simulink model "quad_system_1"  (R2023a)
settings: Solver=VariableStepAuto  StartTime=0.0  StopTime=30  RelTol=1e-7
InitFcn:
  | % Init parameters
  | ax = 0; ay = 0; az = 0;
  | a_theta = 0; a_phi = 0; a_psi = 0;
  | m = 1;
  | J_phi = 1;
  | J_psi = 1;
  | C = 1;
  | L = 1;
  | J_theta = 1;
  | g = 9.81;
  | alpha = 0.9;
  | K = alpha*g;
  | 
  | %Controller for Z/phi
  | k_11 = 100;
  | k_21 = 100;
  | k_12 = 1;
  | k_22 = 1;
  | 
  | %Controller for X/Y
  | k31=100;
  | k41=100;
  | k51=100;
  | k61=10;
  | 
  | k32=100;
  | k42=100;
  | k52=100;
  | k62=10;
  | % k31=1000;
  | % k41=100;
  | % k51=100;
  | % k61=1;
  | %
  | % k32=1000;
  | % k42=100;
  | % k52=100;
  | % k62=1;
  | 
  | J = [0 -1; 1 0];
settings Model: Creator=Dell  LastModifiedBy=Dell
settings DebuggingCC: UnconnectedInputMsg=warning  UnconnectedOutputMsg=warning  UnconnectedLineMsg=warning
settings ModelReferenceCC: EnableRefExpFcnMdlSchedulingChecks=on
settings RTWCC: DLArmComputeVersion=19.05

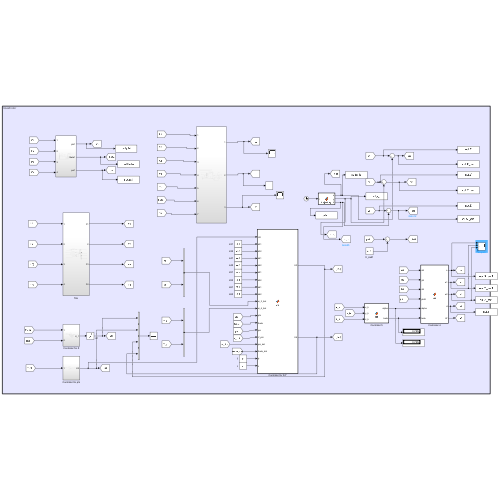
[thumbnail: Simulink's stored preview of the top-level diagram]
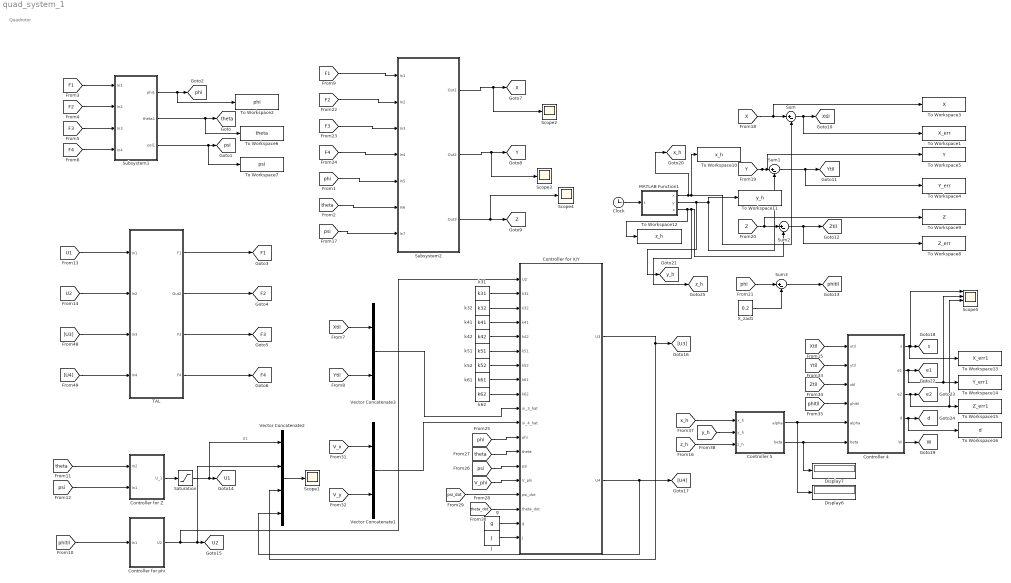
== system quad_system_1 ==
  note: Quadrotor
  Clock : Clock
  Controller 4 : MATLAB Function  TreatAsAtomicUnit=on
  Controller 5 : MATLAB Function  TreatAsAtomicUnit=on
  Controller for X/Y : MATLAB Function  TreatAsAtomicUnit=on
  Controller for Z : Subsystem
  Controller for phi : Subsystem
  Display6 : Display
  Display7 : Display
  J : Constant  Value=J
  MATLAB Function1 : MATLAB Function  TreatAsAtomicUnit=on
  Saturation : Saturate  UpperLimit=K  LowerLimit=-K
  Scope{1..4} (4 alike) : Scope
  Scope5 : Scope  NumInputPorts=4
  Subsystem1 : Subsystem
  Subsystem2 : Subsystem
  Sum{,1..3} (4 alike) : Sum  Inputs=|+-
  TAL : Subsystem
  To Workspace1 : ToWorkspace  VariableName=X_err  SaveFormat=Timeseries  SampleTime=-1
  To Workspace10 : ToWorkspace  VariableName=x_h  SaveFormat=Timeseries  SampleTime=-1
  To Workspace11 : ToWorkspace  VariableName=y_h  SaveFormat=Timeseries  SampleTime=-1
  To Workspace12 : ToWorkspace  VariableName=z_h  SaveFormat=Timeseries  SampleTime=-1
  To Workspace13 : ToWorkspace  VariableName=X_err1  SaveFormat=Timeseries  SampleTime=-1
  To Workspace14 : ToWorkspace  VariableName=Y_err1  SaveFormat=Timeseries  SampleTime=-1
  To Workspace15 : ToWorkspace  VariableName=Z_err1  SaveFormat=Timeseries  SampleTime=-1
  To Workspace16 : ToWorkspace  VariableName=d  SaveFormat=Timeseries  SampleTime=-1
  To Workspace2 : ToWorkspace  VariableName=phi  SaveFormat=Timeseries  SampleTime=-1
  To Workspace3 : ToWorkspace  VariableName=X  SaveFormat=Timeseries  SampleTime=-1
  To Workspace4 : ToWorkspace  VariableName=Y_err  SaveFormat=Timeseries  SampleTime=-1
  To Workspace5 : ToWorkspace  VariableName=Y  SaveFormat=Timeseries  SampleTime=-1
  To Workspace6 : ToWorkspace  VariableName=theta  SaveFormat=Timeseries  SampleTime=-1
  To Workspace7 : ToWorkspace  VariableName=psi  SaveFormat=Timeseries  SampleTime=-1
  To Workspace8 : ToWorkspace  VariableName=Z_err  SaveFormat=Timeseries  SampleTime=-1
  To Workspace9 : ToWorkspace  VariableName=Z  SaveFormat=Timeseries  SampleTime=-1
  Vector Concatenate1 : Concatenate
  Vector Concatenate2 : Concatenate  NumInputs=4
  Vector Concatenate3 : Concatenate
  X_zad1 : Constant  Value=0.2
  g : Constant  Value=g
  k31 : Constant  Value=k31
  k32 : Constant  Value=k32
  k41 : Constant  Value=k41
  k42 : Constant  Value=k42
  k51 : Constant  Value=k51
  k52 : Constant  Value=k52
  k61 : Constant  Value=k61
  k62 : Constant  Value=k62
  tag scope: F1=global, F2=global, F3=global, F4=global, U1=global, U2=global, W=global, X=global, Xtil=global, Y=global, Ytil=global, Z=global, Ztil=global, d=global, e1=global, e2=global, phi=global, phitil=global, psi=global, s=global, theta=global, x_h=global, y_h=global, z_h=global
  wires:
  Subsystem1/1(phi1) -> To Workspace2/1, [phi]
  [phi] -> Subsystem2/5(In5)
  [theta] -> Subsystem2/6(In6)
  [psi] -> Subsystem2/7(In7)
  Subsystem2/2(Out2) -> Scope3/1, [Y]
  Subsystem2/3(Out3) -> Scope4/1, [Z]
  TAL/1(F1) -> [F1]
  TAL/2(Out2) -> [F2]
  TAL/3(F3) -> [F3]
  TAL/4(F4) -> [F4]
  [Z] -> To Workspace9/1, Sum2/1
  [Y] -> To Workspace5/1, Sum1/1
  X_zad1/1 -> Sum3/2
  [phi] -> Sum3/1
  Sum/1 -> To Workspace1/1, [Xtil]
  Sum1/1 -> To Workspace4/1, [Ytil]
  Sum3/1 -> [phitil]
  Sum2/1 -> To Workspace8/1, [Ztil]
  [phitil] -> Controller for phi/1(In1)
  Controller for phi/1(U2) -> Controller for X/Y/1(U2), Vector Concatenate2/2, [U2]
  Controller for Z/1(U_1) -> Saturation/1
  Saturation/1 -> Vector Concatenate2/1, [U1]  "U1"
  [F1] -> Subsystem1/1(In1)
  [F2] -> Subsystem1/2(In2)
  [F3] -> Subsystem1/3(In3)
  [F4] -> Subsystem1/4(In4)
  [F1] -> Subsystem2/1(In1)
  [F2] -> Subsystem2/2(In2)
  [F3] -> Subsystem2/3(In3)
  [F4] -> Subsystem2/4(In4)
  Controller for X/Y/1(U3) -> Vector Concatenate2/3, [U3]
  Controller for X/Y/2(U4) -> Vector Concatenate2/4, [U4]
  [Xtil] -> Vector Concatenate3/1
  [Ytil] -> Vector Concatenate3/2
  [phi] -> Controller for X/Y/12(phi)
  [theta] -> Controller for X/Y/13(theta)
  [psi] -> Controller for X/Y/14(psi)
  [V_phi] -> Controller for X/Y/15(V_phi)
  [psi_dot] -> Controller for X/Y/16(psi_dot)
  [theta_dot] -> Controller for X/Y/17(theta_dot)
  k31/1 -> Controller for X/Y/2(k31)
  k32/1 -> Controller for X/Y/3(k32)
  k41/1 -> Controller for X/Y/4(k41)
  k42/1 -> Controller for X/Y/5(k42)
  g/1 -> Controller for X/Y/18(g)
  J/1 -> Controller for X/Y/19(J)
  Vector Concatenate3/1 -> Controller for X/Y/10(xi_3_hat)
  Vector Concatenate1/1 -> Controller for X/Y/11(xi_4_hat)
  [V_x] -> Vector Concatenate1/1
  [V_y] -> Vector Concatenate1/2
  [U3] -> TAL/3(In3)
  [U4] -> TAL/4(In4)
  [U1] -> TAL/1(In1)
  [U2] -> TAL/2(In2)
  Subsystem2/1(Out1) -> Scope2/1, [X]
  [theta] -> Controller for Z/1(In2)
  [psi] -> Controller for Z/2(In1)
  Vector Concatenate2/1 -> Scope1/1
  [X] -> To Workspace3/1, Sum/1
  k51/1 -> Controller for X/Y/6(k51)
  k52/1 -> Controller for X/Y/7(k52)
  k61/1 -> Controller for X/Y/8(k61)
  k62/1 -> Controller for X/Y/9(k62)
  Subsystem1/2(theta1) -> To Workspace6/1, [theta]
  Subsystem1/3(psi1) -> To Workspace7/1, [psi]
  Clock/1 -> MATLAB Function1/1(t)
  MATLAB Function1/1(x) -> [x_h], To Workspace10/1, Sum/2
  MATLAB Function1/2(y) -> [y_h], Sum1/2, To Workspace11/1
  MATLAB Function1/3(z) -> To Workspace12/1, [z_h], Sum2/2
  Controller 4/3(e2) -> Scope5/3, To Workspace15/1, [e2]
  [Ytil] -> Controller 4/2(ytil)
  [Xtil] -> Controller 4/1(xtil)
  [x_h] -> Controller 5/1(x_h)
  Controller 4/4(d) -> To Workspace16/1, [d]
  [Ztil] -> Controller 4/3(ztil)
  [z_h] -> Controller 5/3(z_h)
  Controller 4/2(e1) -> Scope5/2, To Workspace14/1, [e1]
  [phitil] -> Controller 4/4(phitil)
  [y_h] -> Controller 5/2(y_h)
  Controller 4/5(W) -> [W]
  Controller 5/2(beta) -> Controller 4/6(beta), Display7/1
  Controller 5/1(alpha) -> Display6/1, Controller 4/5(alpha)
  Controller 4/1(s) -> Scope5/1, [s], To Workspace13/1

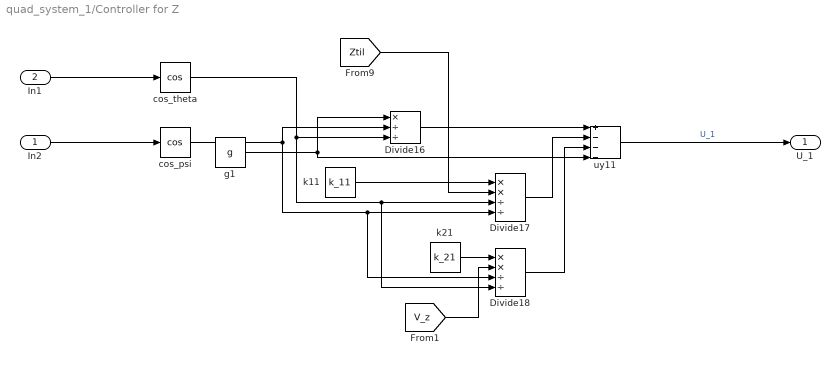
== system quad_system_1/Controller for Z ==
  In2 : Inport
  In1 : Inport  Port=2
  Divide16 : Product  Inputs=*//
  Divide17 : Product  Inputs=**//
  Divide18 : Product  Inputs=**//
  cos_psi : Trigonometry  Operator=cos
  cos_theta : Trigonometry  Operator=cos
  g1 : Constant  Value=g
  k11 : Constant  Value=k_11
  k21 : Constant  Value=k_21
  uy11 : Sum  Inputs=+---
  U_1 : Outport
  wires:
  k11/1 -> Divide17/1
  g1/1 -> uy11/4, Divide16/1
  Divide16/1 -> uy11/1
  k21/1 -> Divide18/1
  Divide18/1 -> uy11/3
  Divide17/1 -> uy11/2
  cos_theta/1 -> Divide16/3, Divide18/4, Divide17/3
  [Ztil] -> Divide17/2
  cos_psi/1 -> Divide16/2, Divide18/3, Divide17/4
  uy11/1 -> U_1/1  "U_1"
  In1/1 -> cos_theta/1
  In2/1 -> cos_psi/1
  [V_z] -> Divide18/2

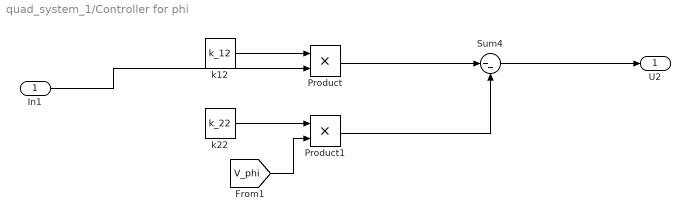
== system quad_system_1/Controller for phi ==
  In1 : Inport
  Product : Product
  Product1 : Product
  Sum4 : Sum  Inputs=|--
  k12 : Constant  Value=k_12
  k22 : Constant  Value=k_22
  U2 : Outport
  wires:
  In1/1 -> Product/2
  Sum4/1 -> U2/1
  k22/1 -> Product1/1
  k12/1 -> Product/1
  Product/1 -> Sum4/1
  Product1/1 -> Sum4/2
  [V_phi] -> Product1/2

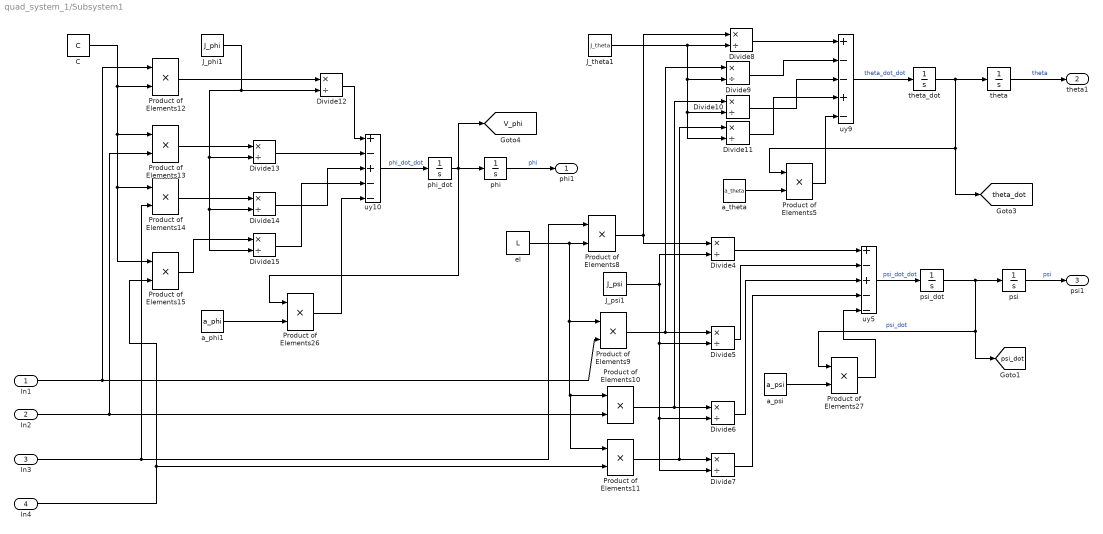
== system quad_system_1/Subsystem1 ==
  In1 : Inport
  In2 : Inport  Port=2
  In3 : Inport  Port=3
  In4 : Inport  Port=4
  C : Constant  Value=C
  Divide{4..15} (12 alike) : Product  Inputs=*/
  J_phi1 : Constant  Value=J_phi
  J_psi1 : Constant  Value=J_psi
  J_theta1 : Constant  Value=J_theta
  Product of Elements{5,8..15,26..27} (11 alike) : Product
  a_phi1 : Constant  Value=a_phi
  a_psi : Constant  Value=a_psi
  a_theta : Constant  Value=a_theta
  el : Constant  Value=L
  phi : Integrator
  phi_dot : Integrator
  psi : Integrator
  psi_dot : Integrator
  theta : Integrator
  theta_dot : Integrator
  uy10 : Sum  Inputs=+-+--
  uy5 : Sum  Inputs=+-+--
  uy9 : Sum  Inputs=+--+-
  phi1 : Outport
  theta1 : Outport  Port=2
  psi1 : Outport  Port=3
  tag scope: V_phi=global, psi_dot=global, theta_dot=global
  wires:
  a_theta/1 -> Product of Elements5/2
  Divide11/1 -> uy9/4
  Product of Elements15/1 -> Divide15/1
  Divide10/1 -> uy9/3
  psi_dot/1 -> [psi_dot], Product of Elements27/1, psi/1  "psi_dot"
  phi/1 -> phi1/1  "phi"
  J_psi1/1 -> Divide4/2, Divide7/2, Divide6/2, Divide5/2
  psi/1 -> psi1/1  "psi"
  Product of Elements8/1 -> Divide4/1, Divide8/1
  In2/1 -> Product of Elements10/2, Product of Elements13/2
  Divide6/1 -> uy5/3
  Product of Elements11/1 -> Divide11/1, Divide7/1
  uy9/1 -> theta_dot/1  "theta_dot_dot"
  theta_dot/1 -> [theta_dot], Product of Elements5/1, theta/1
  J_phi1/1 -> Divide15/2, Divide14/2, Divide13/2, Divide12/2
  C/1 -> Product of Elements15/1, Product of Elements14/1, Product of Elements13/1, Product of Elements12/2
  J_theta1/1 -> Divide11/2, Divide10/2, Divide9/2, Divide8/2
  el/1 -> Product of Elements11/1, Product of Elements10/1, Product of Elements9/1, Product of Elements8/2
  Divide5/1 -> uy5/2
  Divide15/1 -> uy10/4
  Product of Elements9/1 -> Divide5/1, Divide9/1
  Divide13/1 -> uy10/2
  Divide8/1 -> uy9/1
  Divide4/1 -> uy5/1
  Product of Elements13/1 -> Divide13/1
  In4/1 -> Product of Elements15/2, Product of Elements11/2
  Divide9/1 -> uy9/2
  Product of Elements14/1 -> Divide14/1
  Divide7/1 -> uy5/4
  phi_dot/1 -> [V_phi], phi/1, Product of Elements26/1
  Divide14/1 -> uy10/3
  In3/1 -> Product of Elements8/1, Product of Elements14/2
  a_psi/1 -> Product of Elements27/2
  In1/1 -> Product of Elements12/1, Product of Elements9/2
  Product of Elements10/1 -> Divide10/1, Divide6/1
  Divide12/1 -> uy10/1
  uy5/1 -> psi_dot/1  "psi_dot_dot"
  Product of Elements12/1 -> Divide12/1
  Product of Elements5/1 -> uy9/5
  Product of Elements27/1 -> uy5/5
  uy10/1 -> phi_dot/1  "phi_dot_dot"
  Product of Elements26/1 -> uy10/5
  a_phi1/1 -> Product of Elements26/2
  theta/1 -> theta1/1  "theta"

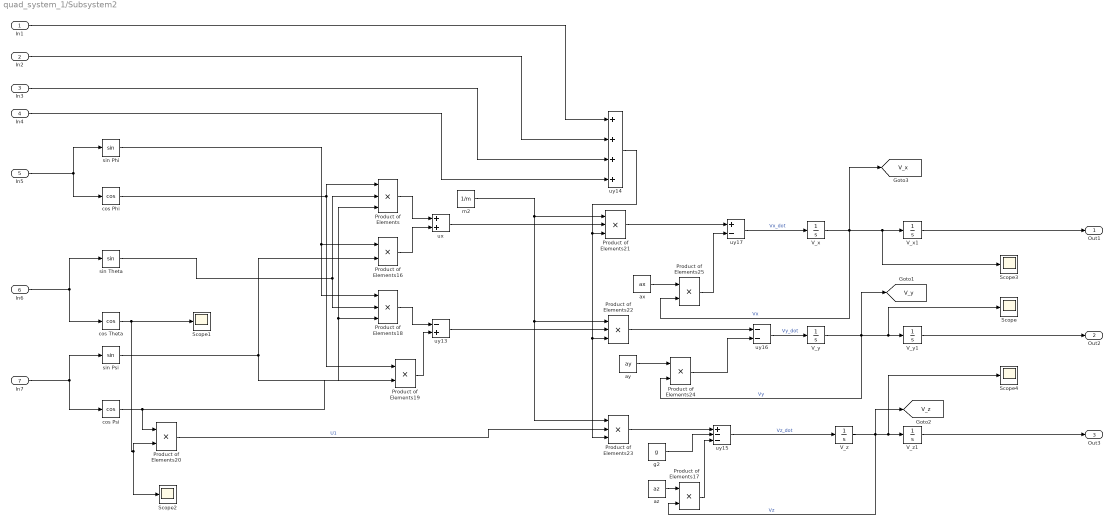
== system quad_system_1/Subsystem2 ==
  In1 : Inport
  In2 : Inport  Port=2
  In3 : Inport  Port=3
  In4 : Inport  Port=4
  In5 : Inport  Port=5
  In6 : Inport  Port=6
  In7 : Inport  Port=7
  Product of Elements{,18,21..23} (5 alike) : Product  Inputs=3
  Product of Elements{16..17,19..20,24..25} (6 alike) : Product
  Scope{,1..4} (5 alike) : Scope
  V_x : Integrator
  V_x1 : Integrator  InitialCondition=2
  V_y : Integrator
  V_y1 : Integrator
  V_z : Integrator
  V_z1 : Integrator
  ax : Constant  Value=ax
  ay : Constant  Value=ay
  az : Constant  Value=az
  cos Phi : Trigonometry  Operator=cos
  cos Psi : Trigonometry  Operator=cos
  cos Theta : Trigonometry  Operator=cos
  g2 : Constant  Value=g
  m2 : Constant  Value=1/m
  sin Phi : Trigonometry
  sin Psi : Trigonometry
  sin Theta : Trigonometry
  ux : Sum
  uy13 : Sum  Inputs=-+
  uy14 : Sum  Inputs=++++
  uy15 : Sum  Inputs=+--
  uy16 : Sum  Inputs=--
  uy17 : Sum  Inputs=+-
  Out1 : Outport
  Out2 : Outport  Port=2
  Out3 : Outport  Port=3
  tag scope: V_x=global, V_y=global, V_z=global
  wires:
  In3/1 -> uy14/3
  uy17/1 -> V_x/1  "Vx_dot"
  Product of Elements16/1 -> ux/2
  cos Psi/1 -> Product of Elements/3, Product of Elements18/3, Product of Elements20/1
  uy14/1 -> Product of Elements23/3, Product of Elements22/3, Product of Elements21/3
  ux/1 -> Product of Elements21/2
  sin Phi/1 -> Product of Elements16/1, Product of Elements18/1
  m2/1 -> Product of Elements21/1, Product of Elements22/1, Product of Elements23/1
  In4/1 -> uy14/4
  In1/1 -> uy14/1
  g2/1 -> uy15/2
  V_z/1 -> [V_z], Scope4/1, V_z1/1, Product of Elements17/2  "Vz"
  ax/1 -> Product of Elements25/1
  sin Theta/1 -> Product of Elements18/2, Product of Elements/2
  In5/1 -> cos Phi/1, sin Phi/1
  cos Phi/1 -> Product of Elements19/1, Product of Elements/1
  Product of Elements25/1 -> uy17/2
  Product of Elements/1 -> ux/1
  Product of Elements22/1 -> uy16/1
  Product of Elements21/1 -> uy17/1
  sin Psi/1 -> Product of Elements19/2, Product of Elements16/2
  Product of Elements19/1 -> uy13/2
  V_x/1 -> [V_x], Scope3/1, V_x1/1, Product of Elements25/2  "Vx"
  V_x1/1 -> Out1/1
  V_y/1 -> [V_y], Scope/1, V_y1/1, Product of Elements24/2  "Vy"
  uy15/1 -> V_z/1  "Vz_dot"
  Product of Elements24/1 -> uy16/2
  In7/1 -> cos Psi/1, sin Psi/1
  Product of Elements17/1 -> uy15/3
  Product of Elements18/1 -> uy13/1
  Product of Elements23/1 -> uy15/1
  ay/1 -> Product of Elements24/1
  uy13/1 -> Product of Elements22/2
  az/1 -> Product of Elements17/1
  uy16/1 -> V_y/1  "Vy_dot"
  cos Theta/1 -> Scope2/1, Product of Elements20/2, Scope1/1
  In6/1 -> cos Theta/1, sin Theta/1
  In2/1 -> uy14/2
  V_z1/1 -> Out3/1
  V_y1/1 -> Out2/1
  Product of Elements20/1 -> Product of Elements23/2  "U1"

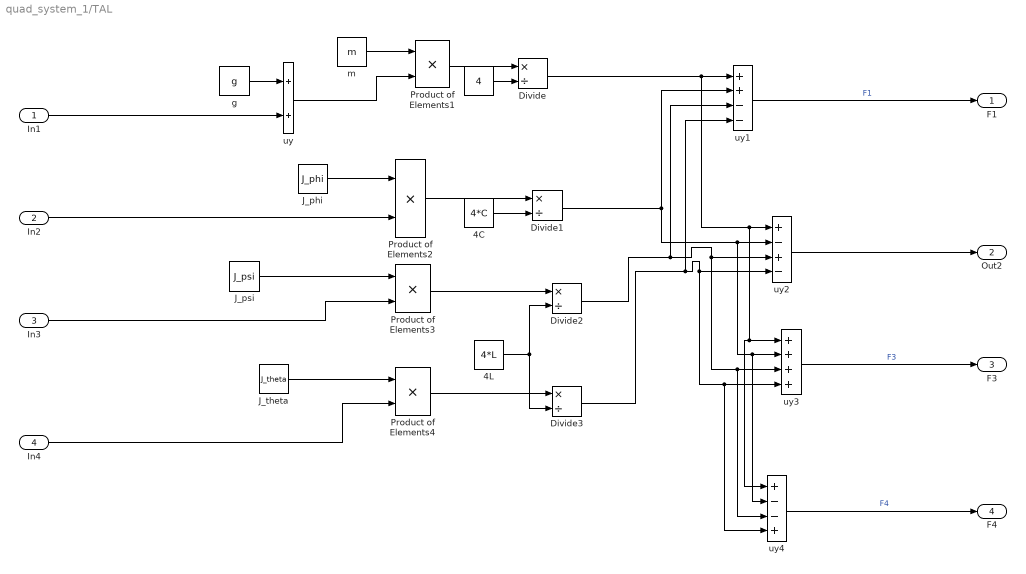
== system quad_system_1/TAL ==
  In1 : Inport
  In2 : Inport  Port=2
  In3 : Inport  Port=3
  In4 : Inport  Port=4
  " " : Constant  Value=4
  4C : Constant  Value=4*C
  4L : Constant  Value=4*L
  Divide{,1..3} (4 alike) : Product  Inputs=*/
  J_phi : Constant  Value=J_phi
  J_psi : Constant  Value=J_psi
  J_theta : Constant  Value=J_theta
  Product of Elements{1..4} (4 alike) : Product
  g : Constant  Value=g
  m : Constant  Value=m
  uy : Sum
  uy1 : Sum  Inputs=++--
  uy2 : Sum  Inputs=+-+-
  uy3 : Sum  Inputs=++++
  uy4 : Sum  Inputs=+--+
  F1 : Outport
  Out2 : Outport  Port=2
  F3 : Outport  Port=3
  F4 : Outport  Port=4
  wires:
  Divide/1 -> uy3/1, uy4/1, uy2/1, uy1/1
  Product of Elements4/1 -> Divide3/1
  In2/1 -> Product of Elements2/2
  Product of Elements1/1 -> Divide/1
  " "/1 -> Divide/2
  Divide1/1 -> uy1/2, uy4/2, uy3/2, uy2/2
  Divide2/1 -> uy4/3, uy3/3, uy2/3, uy1/3
  J_theta/1 -> Product of Elements4/1
  4L/1 -> Divide2/2, Divide3/2
  4C/1 -> Divide1/2
  uy4/1 -> F4/1  "F4"
  Product of Elements3/1 -> Divide2/1
  Divide3/1 -> uy4/4, uy3/4, uy2/4, uy1/4
  uy2/1 -> Out2/1
  In4/1 -> Product of Elements4/2
  J_phi/1 -> Product of Elements2/1
  In3/1 -> Product of Elements3/2
  m/1 -> Product of Elements1/1
  Product of Elements2/1 -> Divide1/1
  g/1 -> uy/1
  uy3/1 -> F3/1  "F3"
  J_psi/1 -> Product of Elements3/1
  uy/1 -> Product of Elements1/2
  uy1/1 -> F1/1  "F1"
  In1/1 -> uy/2

== matlab function quad_system_1/Controller for X//Y ==
  data: U2 input; U3 output; U4 output; k31 input; k32 input; k41 input; k42 input; k51 input; k52 input; k61 input; k62 input; xi_3_hat input; xi_4_hat input; phi input; theta input; psi input; V_phi input; psi_dot input; theta_dot input; g input; J input
function [U3,U4]= fcn(U2, k31, k32, k41, k42, k51, k52, k61, k62, xi_3_hat, xi_4_hat, phi, theta, psi, V_phi, psi_dot, theta_dot, g, J)

b22 = [cos(phi) -sin(phi); sin(phi) cos(phi)]*[-sin(theta)*sin(psi) cos(theta)*cos(psi); -cos(psi) 0];

xi_6_hat = g*[cos(phi) -sin(phi); sin(phi) cos(phi)]*J*[sin(theta)*cos(psi); -sin(psi)]*V_phi+g*[cos(phi) -sin(phi); sin(phi) cos(phi)]*[-sin(theta)*sin(psi) cos(theta)*cos(psi); -cos(psi) 0]*[psi_dot; theta_dot];

xi_5_hat = g*[cos(phi) -sin(phi); sin(phi) cos(phi)]*[sin(theta)*cos(psi); -sin(psi)];

q_2 = J*xi_6_hat*V_phi + g*[cos(phi) -sin(phi); sin(phi) cos(phi)]*[cos(psi) 0; -sin(theta)*sin(psi) cos(theta)*cos(psi)]*[psi_dot; theta_dot]*V_phi + g*[cos(phi) -sin(phi); sin(phi) cos(phi)]*[-2*cos(theta)*sin(psi) -sin(theta)*cos(psi) sin(theta)*cos(psi); 0 sin(psi) 0]*[psi_dot*theta_dot; psi_dot*psi_dot; theta_dot*theta_dot];
b21 = g*J*[cos(phi) -sin(phi); sin(phi) cos(phi)]*[sin(theta)*cos(psi); -sin(psi)];

K3 = diag([k31, k32]); 
K4 = diag([k41, k42]);
K5 = diag([k51, k52]);
K6 = diag([k61, k62]);

U_xy = b22 \ (-q_2 - b21 .* U2 - K3 * xi_3_hat - K4 * xi_4_hat - K5 * xi_5_hat - K6 * xi_6_hat);

U3 = U_xy(1);
U4 = U_xy(2);
end

== matlab function quad_system_1/MATLAB Function1 ==
  data: x output; t input; y output; z output
function [x, y, z] = trajectory(t)
    % Определение ориентиров A, B, C, D
    A = [5, 5, 5];
    B = [10, 10, 5];
    C = [20, 5, 10];
    D = [30, 20, 20];

    % Объединяем ориентиры в матрицу
    waypoints = [A; B; C; D]; 
    % Время достижения ориентиров
    t_waypoints = [5; 10; 20; 30];

    % Интерполяция
    if t < t_waypoints(1)
        % Если время меньше первого ориентира
        x = A(1);
        y = A(2);
        z = A(3);
    elseif t > t_waypoints(end)
        % Если время больше последнего ориентира
        x = D(1);
        y = D(2);
        z = D(3);
    else
        % Линейная интерполяция по x, y и z
        x = interp1(t_waypoints, waypoints(:,1), t, 'linear'); 
        y = interp1(t_waypoints, waypoints(:,2), t, 'linear'); 
        z = interp1(t_waypoints, waypoints(:,3), t, 'linear'); 
    end
end

== matlab function quad_system_1/Controller 4 ==
  data: s output; xtil input; ytil input; ztil input; phitil input; alpha input; beta input; e1 output; e2 output; d output; W output
function [s, e1,e2,d, W]   = fcn(xtil,ytil,ztil,phitil,alpha,beta)

xyzphitil = [xtil;ytil;ztil;phitil];


W=  [cos(beta) 0 sin(beta) 0; 0 1 0 0; -sin(beta) 0 cos(beta) 0; 0 0 0 1]*...
    [cos(alpha) sin(alpha) 0 0; -sin(alpha) cos(alpha) 0 0;  0 0 1 0; 0 0 0 1];


P = W*xyzphitil;

s = P(1);

e1 = P(2);

e2 = P(3);

d = P(4);

zeta =[s;e1;e2;d];

== matlab function quad_system_1/Controller 5 ==
  data: x_h input; y_h input; alpha output; beta output; z_h input
function [alpha,beta]   = fcn(x_h,y_h,z_h)


% atna2(sin *, cos *)

% cos alpha = d varphi_xy / dy;  
% sin alpha = -d varphi_xy / dx;

% cos beta = d varphi_xz / dz;  
% sin beta = -d varphi_xz / dx;


% Прямые x+y = 0 и x+z = 0

alpha = atan2(-(-1), 1);

beta = atan2(-(-1), 1);
